simulink model "VFlexP"  (R2025a)
settings: Solver=ode23tb  StartTime=0.0  StopTime=40  FixedStep=5e-5
model workspace (MAT data in the model file):
  DCop_DCBUCK : object (value not decoded)
  Grid_CCVSC_idx = [2; 3; 4; 5; 6; 7; 8; 9; 10; 11; 12]
  Grid_CCVSCs = 1
  Grid_CCVSCs_buses = 1
  Grid_CCVSCs_toM = [0 1 0 0 0 0 0 0 0 0 0 0 ... (781 elements, 71x11)]
  Grid_C_Lines = [0.1 0.1 0.1 0.1]
  Grid_Cbuses = [0.05000002 0.10000002 0.10000002 0.10000002 0.05000002]
  Grid_DC : object (value not decoded)
  Grid_DCop_DCBUCK : object (value not decoded)
  Grid_DCop_DC_PES : object (value not decoded)
  Grid_DFIGs = 1
  Grid_DFIGs_buses = 1
  Grid_DGs : string (value not decoded)
  Grid_From_buses = [1 2 4 4]
  Grid_GFls = 1
  Grid_GFls_buses = 1
  Grid_GFr_idx = [1; 2; 3]
  Grid_GFrs = 1
  Grid_GFrs_buses = 1
  Grid_GFrs_toM = [1 0 0 0 0 0 0 0 0 1 0 0 ... (15 elements, 5x3)]
  Grid_IG_idx = 1
  Grid_IGs = 1
  Grid_IGs_buses = 1
  Grid_IGs_toM = [1; 0]
  Grid_L_Lines = [0.5 0.5 0.5 0.5]
  Grid_L_Loads = [0.000959999944704 0.000156249997559 0.00154855477548]
  Grid_Lines_fromM : object (value not decoded)
  Grid_Lines_toM : object (value not decoded)
  Grid_Load_buses = [2; 3; 4]
  Grid_Load_busesDC = []
  Grid_MGES_idx = [1; 2; 3]
  Grid_MGESs = 1
  Grid_MGESs_buses = [1; 5; 3]
  Grid_MGESs_toM = [1 0 0 0 0 0 0 0 0 1 0 0 ... (15 elements, 5x3)]
  Grid_MSGs = 1
  Grid_MSGs_buses = 1
  Grid_Nbuses = 5
  Grid_PQ_gen = [3; 2; 2]
  Grid_Ploads = [1250 4000 1250]
  Grid_PloadsDC = []
  Grid_Ps_lf = [0.274439537683 0.78 0.3]
  Grid_Qloads = [0.3 0.5 0.5]
  Grid_Qs_lf = [-0.0366071562958 0.126505596722 -0.0162964024532]
  Grid_R_Lines = [0.01 0.01 0.01 0.01]
  Grid_R_Loads = [3.9999997696 1.24999998047 3.8713869387]
  Grid_R_Loads_DC = 0
  Grid_Rcf = [50000000 50000000 50000000 50000000 50000000]
  Grid_SCs = 1
  Grid_SCs_buses = 1
  Grid_SG_idx = 1
  Grid_SGs = 1
  Grid_SGs_buses = 1
  Grid_SGs_toM = [1; 0]
  Grid_To_buses = [2 3 3 5]
  Grid_VCVSC_idx = [1; 2; 3; 4; 5; 6; 7; 8; 9; 10; 11; 12]
  Grid_VCVSCs = 1
  Grid_VCVSCs_buses = [1; 2; 3; 6; 8; 9; 12; 58; 59; 60; 63; 65]
  Grid_VCVSCs_toM = [1 0 0 0 0 0 0 0 0 0 0 0 ... (852 elements, 71x12)]
  Grid_VSM_idx = [1; 2; 3]
  Grid_VSMs = 1
  Grid_VSMs_buses = 1
  Grid_VSMs_toM = [1 0 0 0 0 0 0 0 0 1 0 0 ... (15 elements, 5x3)]
  Grid_admitt_matrix = [2.15353135314-19.7953135314i  -1.9801980198+19.801980198i; -1.9801980198+19.801980198i  2.15353135314-19.7953135314i]
  Grid_admitt_matrix_noloads = [1.98686468647-19.7953135314i  -1.9801980198+19.801980198i; -1.9801980198+19.801980198i  1.98686468647-19.7953135314i]
  Grid_bus = [1; 2; 6; 7; 8]
  Grid_busDC_complexity = [1 1 1]
  Grid_busDC_complexity_PF = [2 2 2]
  Grid_bus_complexity = [1 1 1 1 1]
  Grid_bus_complexity_PF = [1 1 1 1 1]
  Grid_buses_lf = [1; 5; 3]
  Grid_conductance_matrix = [100.00000002  -100  0; -100  200.00000002  -100; 0  -100  100.00000002]
  Grid_conductance_matrix_noloads = [100.00000002  -100  0; -100  200.00000002  -100; 0  -100  100.00000002]
  Grid_fref : object (value not decoded)
  Grid_gen_static_params : mBase (value not decoded)
  Grid_iPs_lf = [3.64378984326 1.28205128205 3.33333333333]
  Grid_iQs_lf = [-27.3170631425 7.90478860943 -61.3632366329]
  Grid_iadmitt_matrix = [2.88165849328-0.0982918688642i  2.87905051706-0.123273862303i; 2.87905051706-0.123273862303i  2.88165849328-0.0982918688642i]
  Grid_iadmitt_matrix_noloads = [37.5012524798-37.4874983544i  37.4987475202-37.5125016456i; 37.4987475202-37.5125016456i  37.5012524798-37.4874983544i]
  Grid_iconductance_matrix = [16666671.4556  16666671.4489  16666671.4456; 16666671.4489  16666671.4522  16666671.4489; 16666671.4456  16666671.4489  16666671.4556]
  Grid_iconductance_matrix_noloads = [16666671.4556  16666671.4489  16666671.4456; 16666671.4489  16666671.4522  16666671.4489; 16666671.4456  16666671.4489  16666671.4556]
  Grid_init_OK_bool = 1
  Grid_intconv_PF : object (value not decoded)
  Grid_lf_op : op_report (value not decoded)
  Grid_lineDC_complexity = [1 1]
  Grid_lineDC_complexity_PF = [2 2]
  Grid_line_complexity = [1 1 1 1]
  Grid_line_complexity_PF = [3 3 3 3]
  Grid_loadDC_complexity = []
  Grid_loadDC_complexity_PF = []
  Grid_load_complexity = [3 3 3]
  Grid_load_complexity_PF = [4 4 4]
  Grid_opDC_CCVSC : object (value not decoded)
  Grid_opDC_VSM : object (value not decoded)
  Grid_opGFr : object (value not decoded)
  Grid_opVCVSC : object (value not decoded)
  Grid_op_CCVSC : object (value not decoded)
  Grid_op_IG : object (value not decoded)
  Grid_op_MGES : object (value not decoded)
  Grid_op_SG : object (value not decoded)
  Grid_op_VSM : object (value not decoded)
  Grid_shift_lines = [0 0 0 0]
  Grid_tap_lines = [1 1 1 1]
  Grid_v_buses_mod = [1 1 1 0.9837920967 1]
  LinsysParamChangeStruct : Param1 (value not decoded)
  Lline = 0.01
  Rline = 1e-05
  linsys : object (value not decoded)
symbols that are objects in the model workspace (value not decoded): Grid_DCop_DC_PES, Grid_DCop_DCBUCK, Grid_op_CCVSC, Grid_op_IG, Grid_op_MGES, Grid_op_SG, Grid_op_VSM, Grid_opDC_CCVSC, Grid_opDC_VSM, Grid_opGFr, Grid_opVCVSC
undefined symbols (not defined in the file): block_buses_DC, block_idx, CCVSC_idx, Cf, costs, costs2, D, DFIGs_nodes, DiscIntNeverNeededParam, entity, Fb, Fi, From_nodes, grid_linsys, Grid_op_DFIG, Grid_op_DFIG_PQ, Grid_op_MSG, Grid_op_SC, Grid_op_VCVSC, H, initial_states_grid, K_1, K_3, K_5, K_A, K_C, K_IM, K_IR, K_P, K_PM, K_PR, K_S1, K_S2, K_S3, Ki_w, Kic, Kiv, Kp_id, Kp_theta, Kp_w, Kpc, Kpv, last_send, Lc, Lf, Lfd, Lkd1, Lkd2, Lkq1, Lkq2, Lkq3, Lmd, Lmq, Lsd, Lsq, m, M, Matrix_flux_to_i, mp, MSGs_buses ... (+44)
libraries: simulink x1048, eeGeneralControl x12
(part 28 of 50)

== system VFlexP/Grid/Generators/MSG/Stator circuit MSG/Subsystem2 ==
  vad : Inport
  vaq : Inport  Port=2
  id : Inport  Port=3
  iq : Inport  Port=4
  ws : Inport  Port=5
  vd : Inport  Port=6
  vq : Inport  Port=7
  Gain1 : Gain  Gain=Ra_pu
  Gain6 : Gain  Gain=Ra_pu
  Gain7 : Gain  Gain=-1
  Product{1..4} (4 alike) : Product
  Selector1 : Selector  InputPortWidth=length(fref.ref_units)  IndexOptions=Index vector (dialog)  Indices=block_fref  OutputSizes=1
  Sum1 : Sum  Inputs=-|+|-|-  InputSameDT=on  SaturateOnIntegerOverflow=on  OutDataTypeStr=Inherit: Same as first input
  Sum2 : Sum  Inputs=-|+|-|-  InputSameDT=on  SaturateOnIntegerOverflow=on  OutDataTypeStr=Inherit: Same as first input
  psis_d : Integrator  InitialCondition=Grid_op_MSG.op.States(6).x'
  psis_q : Integrator  InitialCondition=Grid_op_MSG.op.States(7).x'
  d : Outport
  q : Outport  Port=2
  wires:
  vaq/1 -> Sum2/3
  Product1/1 -> Sum2/1
  vq/1 -> Sum2/2
  Gain6/1 -> Sum2/4
  vad/1 -> Sum1/4
  vd/1 -> Sum1/2
  ws/1 -> Product1/1, Product2/2
  Product3/1 -> psis_q/1
  Product4/1 -> psis_d/1
  Gain1/1 -> Sum1/1
  psis_q/1 -> Gain7/1, q/1
  id/1 -> Gain1/1
  Product2/1 -> Sum1/3
  iq/1 -> Gain6/1
  Sum1/1 -> Product4/1
  Sum2/1 -> Product3/2
  psis_d/1 -> Product1/2, d/1
  Gain7/1 -> Product2/1
  Selector1/1 -> Product3/1, Product4/2
  [omega_base] -> Selector1/1

== system VFlexP/Grid/Generators/MSG/Subsystem/PI omega ==
  in : Inport
  Gain : Gain  Gain=KPomegar
  Gain1 : Gain  Gain=KIomegar
  Sum : Sum  Inputs=++|
  omegar : Integrator  InitialCondition=Grid_op_MSG.op.States(11).x'
  out : Outport  VectorParamsAs1DForOutWhenUnconnected=off
  wires:
  omegar/1 -> Sum/2
  Gain/1 -> Sum/1
  in/1 -> Gain/1, Gain1/1
  Sum/1 -> out/1
  Gain1/1 -> omegar/1

== system VFlexP/Grid/Generators/MSG/Vc control/PI Vc2 ==
  in : Inport
  Gain : Gain  Gain=Kp_vc2
  Gain1 : Gain  Gain=Ki_vc2
  Sum : Sum  Inputs=++|
  xa3 : Integrator  InitialCondition=Grid_op_MSG.op.States(12).x'
  out : Outport  VectorParamsAs1DForOutWhenUnconnected=off
  wires:
  Gain1/1 -> xa3/1
  Sum/1 -> out/1
  in/1 -> Gain/1, Gain1/1
  Gain/1 -> Sum/1
  xa3/1 -> Sum/2

== system VFlexP/Grid/Generators/SG/Electromagnetic/order 2 ==
  vsd : Inport
  vsq : Inport  Port=2
  ws : Inport  Port=3
  Gain : Gain  Gain=1./Lssd_pu
  Gain1 : Gain  Gain=Rs_pu
  Gain17 : Gain  Gain=-1
  Gain2 : Gain  Gain=Rs_pu
  Gain3 : Gain  Gain=1./Lssd_pu
  Gain4 : Gain
  Gain5 : Gain
  Gain6 : Gain  Gain=-1
  Gain7 : Gain  Gain=-1
  Integrator : Integrator  InitialCondition=Grid_op_SG.op.States(1).x'
  Matrix Concatenate : Concatenate  Mode=Multidimensional array
  Product{1..4} (4 alike) : Product
  Scope : Scope  NumInputPorts=2
      settings: ActiveDisplayYMinimum=-176.647  ActiveDisplayYMaximum=19.6557
  Selector2 : Selector  InputPortWidth=length(fref.ref_units)  IndexOptions=Index vector (dialog)  Indices=block_fref  OutputSizes=1
  Sum : Sum  Inputs=|++
  Sum1 : Sum  Inputs=-|+|-  InputSameDT=on  SaturateOnIntegerOverflow=on  OutDataTypeStr=Inherit: Same as first input
  Sum2 : Sum  Inputs=-|+|-  InputSameDT=on  SaturateOnIntegerOverflow=on  OutDataTypeStr=Inherit: Same as first input
  psis_d : Integrator  InitialCondition=Grid_op_SG.op.States(2).x'
  psis_q : Integrator  InitialCondition=Grid_op_SG.op.States(3).x'
  isd : Outport  VectorParamsAs1DForOutWhenUnconnected=off
  isq : Outport  Port=2  VectorParamsAs1DForOutWhenUnconnected=off
  psi : Outport  Port=3  VectorParamsAs1DForOutWhenUnconnected=off
  wires:
  Product4/1 -> Scope/1, psis_d/1
  vsd/1 -> Sum2/2
  ws/1 -> Product1/1, Product2/2
  Matrix Concatenate/1 -> psi/1
  Product3/1 -> psis_q/1
  Sum1/1 -> Product3/1
  Product1/1 -> Sum2/1
  Product2/1 -> Sum1/3
  Sum2/1 -> Product4/2
  psis_q/1 -> Sum/1, Matrix Concatenate/2, Gain17/1  "psis_q"
  Gain1/1 -> Sum1/1
  [omega_base] -> Selector2/1
  vsq/1 -> Sum1/2
  Gain/1 -> Gain4/1, Gain6/1
  Gain2/1 -> Sum2/3
  Gain3/1 -> Gain5/1, Gain7/1
  Gain17/1 -> Product1/2
  Selector2/1 -> Product4/1, Product3/2
  Sum/1 -> Gain3/1
  Integrator/1 -> Sum/2
  Gain4/1 -> Gain2/1
  Gain5/1 -> Gain1/1
  psis_d/1 -> Product2/1, Matrix Concatenate/1, Gain/1, Scope/2
  Gain6/1 -> isd/1
  Gain7/1 -> isq/1

== system VFlexP/Grid/Generators/SG/Electromagnetic/order 8 ==
  vsd : Inport
  vsq : Inport  Port=2
  vfd : Inport  Port=3
  ws : Inport  Port=4
  Stator circuit : Subsystem
  psi->i : Subsystem
  isd : Outport
  isq : Outport  Port=2
  psi : Outport  Port=3
  wires:
  psi->i/3(isq) -> isq/1
  psi->i/2(i) -> Stator circuit/3(i)
  vsd/1 -> Stator circuit/1(vsd)
  vsq/1 -> Stator circuit/2(vsq)
  ws/1 -> Stator circuit/4(ws)
  Stator circuit/1(psi) -> psi/1, psi->i/1(psi)
  vfd/1 -> Stator circuit/5(vfd)
  psi->i/1(isd) -> isd/1

== system VFlexP/Grid/Generators/SG/Electromagnetic/order 8 nomatrix ==
  vsd : Inport
  vsq : Inport  Port=2
  vfd : Inport  Port=3
  ws : Inport  Port=4
  Assignment : Assignment  NumberOfDimensions=2  DiagnosticForDimensions=Warning  IndexOptions=Index vector (dialog),Assign all  Indices=2,1  OutputSizes=1,1
  Constant : Constant  Value=Lfd_pu  VectorParams1D=off
  Integrator : Integrator  InitialCondition=Grid_op_SG.op.States(5).x'
  Selector : Selector  NumberOfDimensions=2  InputPortWidth=3  IndexOptions=Index vector (dialog),Select all  Indices=2,1  OutputSizes=1,1
  Stator circuit : Subsystem
  Sum3 : Sum  Inputs=++|
  Switch6 : Switch  Criteria=u2 ~= 0  SaturateOnIntegerOverflow=off  InputSameDT=off
  psi->i : Subsystem
  isd : Outport
  isq : Outport  Port=2
  psi : Outport  Port=3
  wires:
  psi->i/3(isq) -> isq/1
  psi->i/2(i) -> Stator circuit/3(i)
  vsd/1 -> Stator circuit/1(vsd)
  vsq/1 -> Stator circuit/2(vsq)
  ws/1 -> Stator circuit/4(ws)
  Stator circuit/1(psi) -> psi/1, Selector/1, Assignment/1
  vfd/1 -> Stator circuit/5(vfd)
  psi->i/1(isd) -> isd/1
  Sum3/1 -> Switch6/3
  Constant/1 -> Switch6/2
  Integrator/1 -> Sum3/2
  Assignment/1 -> psi->i/1(psi)
  Selector/1 -> Sum3/1, Switch6/1
  Switch6/1 -> Assignment/2

== system VFlexP/Grid/Generators/VSM/PC/LPF_P ==
  P : Inport
  Gain : Gain  Gain=100
  I : Integrator  InitialCondition=Grid_op_VSM.op.States(5).x'
  Sum4 : Sum  Inputs=|+-
  P_f : Outport
  wires:
  I/1 -> Sum4/2, P_f/1
  P/1 -> Sum4/1
  Sum4/1 -> Gain/1
  Gain/1 -> I/1

== system VFlexP/Grid/Generators/VSM/PC/LPF_Q ==
  Q : Inport
  Gain : Gain  Gain=10
  I : Integrator  InitialCondition=Grid_op_VSM.op.States(6).x'
  Sum4 : Sum  Inputs=|+-
  Q_f : Outport
  wires:
  Sum4/1 -> Gain/1
  I/1 -> Sum4/2, Q_f/1
  Q/1 -> Sum4/1
  Gain/1 -> I/1

== system VFlexP/Grid/Generators/VSM/PC/Turbine model ==
  In1 : Inport
  Out1 : Outport
  wires:
  In1/1 -> Out1/1

== system VFlexP/Grid/Generators/VSM/PC/WOF_d ==
  In1 : Inport
  Gain : Gain  Gain=10
  Gain1 : Gain  Gain=10
  I : Integrator  InitialConditionSource=external  InitialCondition=Grid_op_VSM.op.States(7).x'
  Sum : Sum  Inputs=+-|
  Sum4 : Sum  Inputs=|+-
  Out1 : Outport
  wires:
  Gain/1 -> I/1
  Sum4/1 -> Gain/1
  In1/1 -> I/2, Sum/1, Sum4/1
  I/1 -> Sum/2, Sum4/2
  Sum/1 -> Gain1/1
  Gain1/1 -> Out1/1

== system VFlexP/Grid/Generators/VSM/RL out/dynamic ==
  v_in_d : Inport
  v_out_d : Inport  Port=2
  v_in_q : Inport  Port=3
  v_out_q : Inport  Port=4
  Gain1 : Gain  Gain=L
  Gain2 : Gain  Gain=R
  Gain3 : Gain  Gain=R
  Gain4 : Gain  Gain=L
  Gain5 : Gain  Gain=invL
  Gain7 : Gain  Gain=invL
  Product{,1..3} (4 alike) : Product
  Selector7 : Selector  InputPortWidth=length(fref.ref_units)  IndexOptions=Index vector (dialog)  Indices=block_fref  OutputSizes=1
  Selector8 : Selector  InputPortWidth=length(fref.ref_units)  IndexOptions=Index vector (dialog)  Indices=block_fref  OutputSizes=1
  Sum4 : Sum  Inputs=+-|
  Sum5 : Sum  Inputs=|-+
  Sum6 : Sum  Inputs=|++
  Sum7 : Sum  Inputs=-+|
  Sum8 : Sum  Inputs=|+-
  Sum9 : Sum  Inputs=-+|
  i_d : Integrator  InitialCondition=Grid_op_VSM.op.States(7).x'
  i_q : Integrator  InitialCondition=Grid_op_VSM.op.States(8).x'
  id : Outport
  iq : Outport  Port=2
  v_outd : Outport  Port=3
  v_outq : Outport  Port=4
  wires:
  v_in_q/1 -> Sum5/2  "v_in_q"
  v_in_d/1 -> Sum4/1  "v_in_d"
  Gain2/1 -> Sum4/2
  i_d/1 -> id/1, Gain1/1, Gain2/1  "id"
  Sum6/1 -> Gain5/1
  [omega_ref] -> Selector7/1  "omega"
  Product/1 -> Sum6/2
  Sum8/1 -> Gain7/1
  Sum4/1 -> Sum7/2
  Product1/1 -> Sum8/2
  Gain4/1 -> Product/1
  Sum7/1 -> Sum6/1
  Gain3/1 -> Sum5/1
  Sum5/1 -> Sum9/2
  i_q/1 -> Gain3/1, Gain4/1, iq/1  "iq"
  Gain1/1 -> Product1/2
  Sum9/1 -> Sum8/1
  v_out_d/1 -> Sum7/1, v_outd/1  "v_out_d"
  v_out_q/1 -> Sum9/1, v_outq/1  "v_out_q"
  Selector7/1 -> Product1/1, Product/2
  [omega_base] -> Selector8/1
  Selector8/1 -> Product2/1, Product3/2
  Product3/1 -> i_d/1
  Gain5/1 -> Product3/1
  Product2/1 -> i_q/1
  Gain7/1 -> Product2/2

== system VFlexP/Grid/Generators/VSM/RL out/static ==
  v_in_d : Inport
  v_out_d : Inport  Port=2
  v_in_q : Inport  Port=3
  v_out_q : Inport  Port=4
  Constant : Constant  Value=R.^2
  Constant1 : Constant
  Divide : Product  Inputs=*/
  Gain : Gain  Gain=L
  Gain1 : Gain  Gain=R
  Gain2 : Gain  Gain=R
  Product{,1..5} (6 alike) : Product
  Selector7 : Selector  InputPortWidth=length(fref.ref_units)  IndexOptions=Index vector (dialog)  Indices=block_fref  OutputSizes=1
  Sum : Sum  Inputs=|++
  Sum1 : Sum  Inputs=|+-
  Sum2 : Sum  Inputs=|+-
  Sum3 : Sum  Inputs=|++
  Sum4 : Sum  Inputs=|-+
  id : Outport
  iq : Outport  Port=2
  v_outd : Outport  Port=3
  v_outq : Outport  Port=4
  wires:
  v_in_q/1 -> Sum2/1  "v_in_q"
  v_out_d/1 -> Sum1/2, v_outd/1  "v_out_d"
  Sum/1 -> Divide/2
  Gain2/1 -> Product5/2
  Product/1 -> Sum/2
  Product1/1 -> Sum3/1
  Product5/1 -> Sum4/2
  Constant/1 -> Sum/1
  Sum2/1 -> Product3/2, Product5/1  "vq"
  Gain/1 -> Product2/2, Product/1, Product/2
  Constant1/1 -> Divide/1
  Product3/1 -> Sum3/2
  Sum1/1 -> Product4/1, Product1/1  "vd"
  Divide/1 -> Product2/1, Gain1/1, Gain2/1
  Product4/1 -> Sum4/1
  Product2/1 -> Product3/1, Product4/2
  Gain1/1 -> Product1/2
  Sum3/1 -> id/1  "id"
  Sum4/1 -> iq/1  "iq"
  v_out_q/1 -> Sum2/2, v_outq/1  "v_out_q"
  v_in_d/1 -> Sum1/1  "v_in_d"
  [omega_ref] -> Selector7/1  "omega"
  Selector7/1 -> Gain/1

== system VFlexP/Grid/Generators/VSM/RL out/static_omega ==
  v_in_d : Inport
  v_out_d : Inport  Port=2
  v_in_q : Inport  Port=3
  v_out_q : Inport  Port=4
  Gain : Gain  Gain=1./(R.^2+L.^2)
  Gain2 : Gain  Gain=1./(R.^2+L.^2)
  Gain3 : Gain  Gain=R
  Gain4 : Gain  Gain=L
  Gain5 : Gain  Gain=L
  Gain6 : Gain  Gain=R
  Sum : Sum  Inputs=|++
  Sum1 : Sum  Inputs=|+-
  Sum2 : Sum  Inputs=|+-
  Sum3 : Sum  Inputs=|-+
  id : Outport
  iq : Outport  Port=2
  v_outd : Outport  Port=3
  v_outq : Outport  Port=4
  wires:
  Gain6/1 -> Sum3/2
  Sum3/1 -> iq/1
  Gain5/1 -> Sum3/1
  Sum/1 -> id/1
  Gain2/1 -> Gain4/1, Gain6/1
  Gain4/1 -> Sum/2
  Gain3/1 -> Sum/1
  Gain/1 -> Gain3/1, Gain5/1
  Sum2/1 -> Gain2/1  "vq"
  Sum1/1 -> Gain/1  "vd"
  v_out_d/1 -> Sum1/2, v_outd/1  "v_out_d"
  v_out_q/1 -> Sum2/2, v_outq/1  "v_out_q"
  v_in_d/1 -> Sum1/1  "v_in_d"
  v_in_q/1 -> Sum2/1  "v_in_q"

== system VFlexP/Grid/Generators/VSM/VCC/dynamic ==
  vodref : Inport
  voqref : Inport  Port=2
  iod : Inport  Port=3
  ioq : Inport  Port=4
  omega : Inport  Port=5
  Cf : Gain  Gain=Cfi
  Cf 1 : Gain  Gain=Cfi
  Fi : Gain  Gain=Fi
  Fi2 : Gain  Gain=Fi
  "Lf " : Gain  Gain=Lf
  Lf1 : Gain  Gain=Lf
  Product{,1..3} (4 alike) : Product
  RC : Subsystem  Variant=on  VariantControlMode=label  LabelModeActiveChoice=dynamic  mask{dynamic=Dynamic, R=Rcf, C=Cfi, fbase=50}
      mask prompts: dynamic "Dynamic behavior"; R "Parallel resistance (p.u.)"; C "Capacitance (p.u.)"; fbase "Base frequency (Hz)"
      mask init: same as VFlexP/Grid/DCAC converters/DC_VCVSC/VCC/dynamic/RC
      mask TypeOptions dynamic: Dynamic | Static | Static omega
  RL : Subsystem  Variant=on  VariantControlMode=label  LabelModeActiveChoice=dynamic  mask(Line){dynamic=Dynamic, R=Rf, L=Lf, fbase=50}
      mask prompts: dynamic "Dynamic behavior"; R "Series resistance (p.u.)"; L "Inductance (p.u.)"; fbase "Base frequency (Hz)"
      mask init: same as VFlexP/Grid/DCAC converters/DC_VCVSC/RL out
      mask Help: web('Documentation/RL.html')
      mask TypeOptions dynamic: Static | Dynamic | Static omega
  Subsystem : Subsystem
  Subsystem1 : Subsystem
  Subsystem2 : Subsystem
  Subsystem3 : Subsystem
  Sum1 : Sum  Inputs=++|
  Sum2 : Sum  Inputs=-+|
  Sum{3,5..6,9} (4 alike) : Sum  Inputs=|++
  Sum4 : Sum  Inputs=++|
  Sum8 : Sum  Inputs=-+|
  vidref : Outport
  viqref : Outport  Port=2
  wires:
  Sum6/1 -> RL/3(v_in_q)
  Sum1/1 -> RL/1(v_in_d)
  Sum9/1 -> Sum6/1  "viqref"
  Sum8/1 -> Sum1/2  "vidref"
  RL/2(iq) -> "Lf "/1, Subsystem3/2(y), RC/3(i_q_in)
  RL/1(id) -> RC/1(i_d_in), Lf1/1, Subsystem2/2(y)
  RC/1(v_d) -> Cf 1/1, Subsystem/2(y), RL/2(v_out_d), Sum1/1, vidref/1
  [omega] -> Product1/1
  omega/1 -> [omega], Product2/1  "omega"
  Subsystem3/1(Out1) -> Sum9/1
  Subsystem2/1(Out1) -> Sum8/2
  Subsystem1/1(Out1) -> Sum3/1
  Subsystem/1(Out1) -> Sum2/2
  Fi2/1 -> Sum5/2
  ioq/1 -> Fi2/1, RC/4(i_q_out)  "ioq"
  [omega] -> Product3/1, RC/5(omega)  "omega"
  Sum3/1 -> Sum5/1
  "Lf "/1 -> Product/1
  Sum2/1 -> Sum4/2
  iod/1 -> Fi/1, RC/2(i_d_out)  "iod"
  Product1/1 -> Sum2/1
  Sum4/1 -> Subsystem2/1(ref)  "ildref"
  Cf/1 -> Product1/2
  Cf 1/1 -> Product2/2
  Product2/1 -> Sum3/2
  Product3/1 -> Sum9/2
  voqref/1 -> Subsystem1/1(ref)  "voqref"
  Fi/1 -> Sum4/1
  Lf1/1 -> Product3/2
  [omega] -> Product/2
  RC/2(v_q) -> Cf/1, Subsystem1/2(y), RL/4(v_out_q), Sum6/2, viqref/1  "voq"
  vodref/1 -> Subsystem/1(ref)  "vodref"
  Product/1 -> Sum8/1
  Sum5/1 -> Subsystem3/1(ref)  "ilqref"

== system VFlexP/Grid/Generators/VSM/VCC/dynamic_VC ==
  vodref : Inport
  voqref : Inport  Port=2
  iod : Inport  Port=3
  ioq : Inport  Port=4
  omega : Inport  Port=5
  Cf : Gain  Gain=Cfi
  Cf 1 : Gain  Gain=Cfi
  Fi : Gain  Gain=Fi
  Fi2 : Gain  Gain=Fi
  Product1 : Product
  Product2 : Product
  RC : Subsystem  Variant=on  VariantControlMode=label  LabelModeActiveChoice=dynamic  mask{dynamic=Dynamic, R=Rcf, C=Cfi, fbase=Fb}
      mask prompts: dynamic "Dynamic behavior"; R "Parallel resistance (p.u.)"; C "Capacitance (p.u.)"; fbase "Base frequency (Hz)"
      mask init: same as VFlexP/Grid/DCAC converters/DC_VCVSC/VCC/dynamic/RC
      mask TypeOptions dynamic: Dynamic | Static | Static omega
  Subsystem : Subsystem
  Subsystem1 : Subsystem
  Sum2 : Sum  Inputs=-+|
  Sum3 : Sum  Inputs=|++
  Sum4 : Sum  Inputs=++|
  Sum5 : Sum  Inputs=|++
  vidref : Outport
  viqref : Outport  Port=2
  wires:
  Sum5/1 -> RC/3(i_q_in)
  Sum4/1 -> RC/1(i_d_in)
  RC/1(v_d) -> Subsystem/2(y), Cf 1/1, vidref/1
  vodref/1 -> Subsystem/1(ref)  "vodref"
  RC/2(v_q) -> Subsystem1/2(y), Cf/1, viqref/1
  Fi/1 -> Sum4/1
  voqref/1 -> Subsystem1/1(ref)  "voqref"
  Product2/1 -> Sum3/2
  Cf 1/1 -> Product2/2
  Cf/1 -> Product1/2
  Product1/1 -> Sum2/1
  iod/1 -> Fi/1, RC/2(i_d_out)  "iod"
  Sum2/1 -> Sum4/2
  Sum3/1 -> Sum5/1
  ioq/1 -> Fi2/1, RC/4(i_q_out)  "ioq"
  Fi2/1 -> Sum5/2
  Subsystem/1(Out1) -> Sum2/2
  Subsystem1/1(Out1) -> Sum3/1
  omega/1 -> [omega], Product2/1, RC/5(omega)  "omega"
  [omega] -> Product1/1

== system VFlexP/Grid/Generators/VSM/VCC/dynamic_limiting ==
  note: Current limiting, no priority
  vodref : Inport
  voqref : Inport  Port=2
  iod : Inport  Port=3
  ioq : Inport  Port=4
  omega : Inport  Port=5
  Abs : Abs  ZeroCross=off  SaturateOnIntegerOverflow=off
  Abs1 : Abs  ZeroCross=off  SaturateOnIntegerOverflow=off
  Abs2 : Abs  ZeroCross=off  SaturateOnIntegerOverflow=off
  Cf : Gain  Gain=Cfi
  Cf 1 : Gain  Gain=Cfi
  Divide : Product  Inputs=*/
  Divide1 : Product  Inputs=*/
  Fi : Gain  Gain=Fi
  Fi2 : Gain  Gain=Fi
  Gain : Gain  Gain=-1
  Gain1 : Gain  Gain=-1
  "Lf " : Gain  Gain=Lf
  Lf1 : Gain  Gain=Lf
  Memory : Memory  InitialCondition=1  LinearizeMemory=on
  Memory1 : Memory  InitialCondition=1  LinearizeMemory=on
  PIi_d : Subsystem
  PIi_q : Subsystem
  PIv_d : Subsystem
  PIv_q : Subsystem
  Product{,1..3} (4 alike) : Product
  RC : Subsystem  Variant=on  VariantControlMode=label  LabelModeActiveChoice=dynamic  mask{dynamic=Dynamic, R=Rcf, C=Cfi, fbase=Fb}
      mask prompts: dynamic "Dynamic behavior"; R "Parallel resistance (p.u.)"; C "Capacitance (p.u.)"; fbase "Base frequency (Hz)"
      mask init: same as VFlexP/Grid/DCAC converters/DC_VCVSC/VCC/dynamic/RC
      mask TypeOptions dynamic: Dynamic | Static | Static omega
  RL : Subsystem  Variant=on  VariantControlMode=label  LabelModeActiveChoice=dynamic  mask(Line){dynamic=Dynamic, R=Rf, L=Lf, fbase=Fb}
      mask prompts: dynamic "Dynamic behavior"; R "Series resistance (p.u.)"; L "Inductance (p.u.)"; fbase "Base frequency (Hz)"
      mask init: same as VFlexP/Grid/DCAC converters/DC_VCVSC/RL out
      mask Help: web('Documentation/RL.html')
      mask TypeOptions dynamic: Static | Dynamic | Static omega
  Real-Imag to Complex : RealImagToComplex
  Relational Operator : RelationalOperator  Operator===  OutDataTypeStr=boolean  ZeroCross=off  RndMeth=Simplest  InputSameDT=off
  Relational Operator1 : RelationalOperator  Operator===  OutDataTypeStr=boolean  ZeroCross=off  RndMeth=Simplest  InputSameDT=off
  Saturation Dynamic : simulink/Discontinuities/Saturation Dynamic  OutMin=[]  OutMax=[]  OutDataTypeStr=Inherit: Same as second input  OutDataType=fixdt(1, 16)  OutScaling=2^-10  DoSatur=off
  Saturation Dynamic1 : simulink/Discontinuities/Saturation Dynamic  OutMin=[]  OutMax=[]  OutDataTypeStr=Inherit: Same as second input  OutDataType=fixdt(1, 16)  OutScaling=2^-10  DoSatur=off
  Sum : Sum  Inputs=|+-
  Sum{1..2,6,8} (4 alike) : Sum  Inputs=-+|
  Sum3 : Sum  Inputs=|++
  Sum4 : Sum  Inputs=++|
  Sum5 : Sum  Inputs=|++
  Sum7 : Sum  Inputs=|+-
  Sum9 : Sum  Inputs=|++
  vidref : Outport
  viqref : Outport  Port=2
  wires:
  Memory/1 -> PIv_d/2(In2)
  Memory1/1 -> PIv_q/2(In2)
  Relational Operator1/1 -> Memory1/1
  Sum/1 -> PIv_q/1(In1)
  Relational Operator/1 -> Memory/1
  Sum1/1 -> PIv_d/1(In1)
  Gain1/1 -> Saturation Dynamic/3
  Gain/1 -> Saturation Dynamic1/3
  Divide1/1 -> Saturation Dynamic1/1, Gain/1
  Divide/1 -> Saturation Dynamic/1, Gain1/1
  Abs/1 -> Divide/2, Divide1/2
  Real-Imag to Complex/1 -> Abs/1
  Sum5/1 -> Real-Imag to Complex/2, Saturation Dynamic1/2, Abs1/1, Relational Operator1/1  "ilqref"
  Product/1 -> Sum8/1
  vodref/1 -> Sum1/2  "vodref"
  RC/2(v_q) -> viqref/1, RL/4(v_out_q), Sum/2, Cf/1  "voq"
  [omega] -> Product/2
  Lf1/1 -> Product3/2
  Fi/1 -> Sum4/1
  Sum6/1 -> PIi_d/1(In1)
  voqref/1 -> Sum/1  "voqref"
  Product3/1 -> Sum9/2
  Product2/1 -> Sum3/2
  Cf 1/1 -> Product2/2
  Cf/1 -> Product1/2
  Sum4/1 -> Real-Imag to Complex/1, Saturation Dynamic/2, Abs2/1, Relational Operator/1  "ildref"
  Product1/1 -> Sum2/1
  iod/1 -> RC/2(i_d_out), Fi/1  "iod"
  Sum2/1 -> Sum4/2
  Sum7/1 -> PIi_q/1(In1)
  "Lf "/1 -> Product/1
  Sum3/1 -> Sum5/1
  [omega] -> RC/5(omega), Product3/1  "omega"
  ioq/1 -> RC/4(i_q_out), Fi2/1  "ioq"
  Fi2/1 -> Sum5/2
  PIv_d/1(Out1) -> Sum2/2
  PIv_q/1(Out1) -> Sum3/1
  PIi_d/1(Out1) -> Sum8/2
  PIi_q/1(Out1) -> Sum9/1
  omega/1 -> Product2/1, [omega]  "omega"
  [omega] -> Product1/1
  RC/1(v_d) -> vidref/1, RL/2(v_out_d), Cf 1/1, Sum1/1
  RL/1(id) -> Lf1/1, Sum6/1, RC/1(i_d_in)
  RL/2(iq) -> RC/3(i_q_in), "Lf "/1, Sum7/2
  Sum8/1 -> RL/1(v_in_d)  "vidref"
  Sum9/1 -> RL/3(v_in_q)  "viqref"
  Abs1/1 -> Divide1/1
  Abs2/1 -> Divide/1
  Saturation Dynamic1/1 -> Relational Operator1/2, Sum7/1
  Saturation Dynamic/1 -> Relational Operator/2, Sum6/2

== system VFlexP/Grid/Generators/VSM/VCC/static ==
  vodref : Inport
  voqref : Inport  Port=2
  iod : Inport  Port=3
  ioq : Inport  Port=4
  omega : Inport  Port=5
  Terminator : Terminator
  Terminator1 : Terminator
  Terminator2 : Terminator
  vidref : Outport
  viqref : Outport  Port=2
  wires:
  omega/1 -> Terminator2/1  "ioq"
  ioq/1 -> Terminator1/1  "ioq"
  iod/1 -> Terminator/1  "iod"
  vodref/1 -> vidref/1  "vodref"
  voqref/1 -> viqref/1  "voqref"

== system VFlexP/Grid/Generators/VSM/VI/WOF_d ==
  In1 : Inport
  Gain : Gain  Gain=iTf
  I : Integrator  InitialConditionSource=external  InitialCondition=Grid_op_VCVSC.op.States(6).x'
  Sum : Sum  Inputs=+-|
  Sum4 : Sum  Inputs=|+-
  Out1 : Outport
  wires:
  Gain/1 -> I/1
  Sum4/1 -> Gain/1
  In1/1 -> I/2, Sum/1, Sum4/1
  I/1 -> Sum/2, Sum4/2
  Sum/1 -> Out1/1

== system VFlexP/Grid/Generators/VSM/VI/WOF_q ==
  In1 : Inport
  Gain : Gain  Gain=iTf
  I : Integrator  InitialConditionSource=external  InitialCondition=Grid_op_VCVSC.op.States(7).x'
  Sum : Sum  Inputs=+-|
  Sum4 : Sum  Inputs=|+-
  Out1 : Outport
  wires:
  Gain/1 -> I/1
  Sum4/1 -> Gain/1
  In1/1 -> I/2, Sum/1, Sum4/1
  I/1 -> Sum/2, Sum4/2
  Sum/1 -> Out1/1

== system VFlexP/Grid/Grid/Dynamic/Buses/dynamic ==
  i_in : Inport
  i_out : Inport  Port=2
  Constant : Constant  Value=zeros(1, sum(bus_complexity == 1))  VectorParams1D=off
  Divide : Product  Inputs=*/
  Divide1 : Product  Inputs=*/
  For Each Subsystem : Subsystem  TreatAsAtomicUnit=on
  Gain1 : Gain  Gain=1./Rcf(bus_complexity == 1)
  Gain2 : Gain  Gain=1./Rcf(bus_complexity == 1)
  Matrix Concatenate : Concatenate  NumInputs=3  Mode=Multidimensional array
  Product : Product  Inputs=3
  Product1 : Product  Inputs=3
  Product2 : Product
  Product3 : Product
  Selector : Selector  NumberOfDimensions=2  InputPortWidth=3  IndexOptions=Index vector (dialog),Index vector (dialog)  Indices=1,find(bus_complexity == 1)  OutputSizes=1,1
  Selector1 : Selector  NumberOfDimensions=2  InputPortWidth=3  IndexOptions=Index vector (dialog),Index vector (dialog)  Indices=2,find(bus_complexity == 1)  OutputSizes=1,1
  Selector2 : Selector  NumberOfDimensions=2  InputPortWidth=3  IndexOptions=Index vector (dialog),Index vector (dialog)  Indices=1,find(bus_complexity == 1)  OutputSizes=1,1
  Selector3 : Selector  NumberOfDimensions=2  InputPortWidth=3  IndexOptions=Index vector (dialog),Index vector (dialog)  Indices=2,find(bus_complexity == 1)  OutputSizes=1,1
  Selector4 : Selector  InputPortWidth=length(fref.ref_units)  IndexOptions=Index vector (dialog)  Indices=fref.buses(bus_complexity == 1)  OutputSizes=1
  Selector5 : Selector  InputPortWidth=length(Cbuses)  IndexOptions=Index vector (dialog)  Indices=find(bus_complexity == 1)  OutputSizes=1
  Selector8 : Selector  InputPortWidth=length(fref.ref_units)  IndexOptions=Index vector (dialog)  Indices=fref.buses(bus_complexity == 1)  OutputSizes=1
  Signal Specification : SignalSpecification  Dimensions=[3 sum(bus_complexity == 1)]
  Sum10 : Sum  Inputs=|-++
  Sum11 : Sum  Inputs=-+|
  Sum12 : Sum  Inputs=|+-
  Sum13 : Sum  Inputs=-+-|
  vd : Integrator  InitialCondition=Grid_lf_op.op_report.Outputs(7).y(bus_complexity == 1)
  vq : Integrator  InitialCondition=Grid_lf_op.op_report.Outputs(8).y(bus_complexity == 1)
  v : Outport
  wires:
  Sum10/1 -> Divide/1
  vq/1 -> Product1/1, Gain2/1, Matrix Concatenate/2  "vq"
  Product1/1 -> Sum10/3
  Gain2/1 -> Sum13/3
  Product/1 -> Sum13/1
  Sum11/1 -> Sum10/2
  [omega_ref] -> Selector4/1  "omega"
  Gain1/1 -> Sum10/1
  Sum12/1 -> Sum13/2
  vd/1 -> Gain1/1, Matrix Concatenate/1, Product/1  "vd"
  Selector/1 -> Sum11/2  "id1"
  Selector2/1 -> Sum11/1  "id2"
  Selector1/1 -> Sum12/1  "iq1"
  Selector3/1 -> Sum12/2  "iq2"
  i_in/1 -> Selector/1, Selector1/1
  i_out/1 -> Selector3/1, Selector2/1
  Matrix Concatenate/1 -> Signal Specification/1
  For Each Subsystem/1(Out1) -> v/1
  Signal Specification/1 -> For Each Subsystem/1(In1)
  Constant/1 -> Matrix Concatenate/3
  Selector4/1 -> Product1/2, Product/2
  Divide/1 -> Product2/1
  Divide1/1 -> Product3/2
  [omega_base] -> Selector8/1
  Selector8/1 -> Product2/2, Product3/1
  Product2/1 -> vd/1
  Product3/1 -> vq/1
  [Cbuses] -> Selector5/1
  Selector5/1 -> [Cb]
  [Cb] -> Product/3
  [Cb] -> Product1/3
  [Cb] -> Divide/2
  [Cb] -> Divide1/2
  Sum13/1 -> Divide1/1

== system VFlexP/Grid/Grid/Dynamic/Buses/only R ==
  i_in : Inport
  i_out : Inport  Port=2
  Constant : Constant  Value=zeros(1, sum(bus_complexity == 4))  VectorParams1D=off
  For Each Subsystem : Subsystem  TreatAsAtomicUnit=on
  Gain : Gain  Gain=Rcf(bus_complexity == 4)
  Gain2 : Gain  Gain=Rcf(bus_complexity == 4)
  Matrix Concatenate : Concatenate  NumInputs=3  Mode=Multidimensional array
  Selector : Selector  NumberOfDimensions=2  InputPortWidth=3  IndexOptions=Index vector (dialog),Index vector (dialog)  Indices=1,find(bus_complexity == 4)  OutputSizes=1,1
  Selector1 : Selector  NumberOfDimensions=2  InputPortWidth=3  IndexOptions=Index vector (dialog),Index vector (dialog)  Indices=2,find(bus_complexity == 4)  OutputSizes=1,1
  Selector2 : Selector  NumberOfDimensions=2  InputPortWidth=3  IndexOptions=Index vector (dialog),Index vector (dialog)  Indices=1,find(bus_complexity == 4)  OutputSizes=1,1
  Selector3 : Selector  NumberOfDimensions=2  InputPortWidth=3  IndexOptions=Index vector (dialog),Index vector (dialog)  Indices=2,find(bus_complexity == 4)  OutputSizes=1,1
  Sum1 : Sum  Inputs=|+-
  Sum2 : Sum  Inputs=|+-
  v : Outport
  wires:
  Selector1/1 -> Sum2/1  "iq1"
  Sum1/1 -> Gain/1  "id"
  Sum2/1 -> Gain2/1  "iq"
  Selector3/1 -> Sum2/2  "iq2"
  Selector/1 -> Sum1/1  "id"
  Selector2/1 -> Sum1/2
  Gain2/1 -> Matrix Concatenate/2
  Gain/1 -> Matrix Concatenate/1
  i_in/1 -> Selector/1, Selector1/1
  Matrix Concatenate/1 -> For Each Subsystem/1(In1)
  i_out/1 -> Selector2/1, Selector3/1
  For Each Subsystem/1(Out1) -> v/1
  Constant/1 -> Matrix Concatenate/3

== system VFlexP/Grid/Grid/Dynamic/Buses/static ==
  i_in : Inport
  i_out : Inport  Port=2
  Constant : Constant  Value=(1./Rcf(bus_complexity == 2)).^2  VectorParams1D=off
  Constant1 : Constant
  Constant2 : Constant  Value=zeros(1, sum(bus_complexity == 2))  VectorParams1D=off
  Divide : Product  Inputs=*/
  For Each Subsystem : Subsystem  TreatAsAtomicUnit=on
  Gain1 : Gain  Gain=1./Rcf(bus_complexity == 2)
  Gain2 : Gain  Gain=1./Rcf(bus_complexity == 2)
  Matrix Concatenate : Concatenate  NumInputs=3  Mode=Multidimensional array
  Product{,1..6} (7 alike) : Product
  Selector : Selector  NumberOfDimensions=2  InputPortWidth=3  IndexOptions=Index vector (dialog),Index vector (dialog)  Indices=1,find(bus_complexity == 2)  OutputSizes=1,1
  Selector1 : Selector  NumberOfDimensions=2  InputPortWidth=3  IndexOptions=Index vector (dialog),Index vector (dialog)  Indices=2,find(bus_complexity == 2)  OutputSizes=1,1
  Selector2 : Selector  NumberOfDimensions=2  InputPortWidth=3  IndexOptions=Index vector (dialog),Index vector (dialog)  Indices=1,find(bus_complexity == 2)  OutputSizes=1,1
  Selector3 : Selector  NumberOfDimensions=2  InputPortWidth=3  IndexOptions=Index vector (dialog),Index vector (dialog)  Indices=2,find(bus_complexity == 2)  OutputSizes=1,1
  Selector4 : Selector  InputPortWidth=length(fref.ref_units)  IndexOptions=Index vector (dialog)  Indices=fref.buses(bus_complexity == 2)  OutputSizes=1
  Selector5 : Selector  InputPortWidth=length(Cbuses)  IndexOptions=Index vector (dialog)  Indices=find(bus_complexity == 2)  OutputSizes=1
  Sum : Sum  Inputs=|++
  Sum1 : Sum  Inputs=|-+
  Sum2 : Sum  Inputs=|+-
  Sum3 : Sum  Inputs=|++
  Sum4 : Sum  Inputs=|-+
  v : Outport
  wires:
  Product5/1 -> Sum4/2
  Gain2/1 -> Product5/2
  Product4/1 -> Sum4/1
  Product2/1 -> Product3/1, Product4/2
  Product3/1 -> Sum3/2
  Product1/1 -> Sum3/1
  Divide/1 -> Product2/1, Gain1/1, Product5/1
  Gain1/1 -> Product1/2
  Sum2/1 -> Product3/2, Gain2/1  "iq"
  Sum1/1 -> Product4/1, Product1/1  "id"
  Constant1/1 -> Divide/1
  Product/1 -> Sum/2
  Product6/1 -> Product/1, Product/2, Product2/2
  Sum/1 -> Divide/2
  Constant/1 -> Sum/1
  Sum4/1 -> Matrix Concatenate/2  "vq"
  Sum3/1 -> Matrix Concatenate/1  "vd"
  [omega_ref] -> Selector4/1  "omega"
  Selector/1 -> Sum1/2  "id1"
  Selector2/1 -> Sum1/1  "id2"
  Selector1/1 -> Sum2/1  "iq1"
  Selector3/1 -> Sum2/2  "iq2"
  i_in/1 -> Selector/1, Selector1/1
  Matrix Concatenate/1 -> For Each Subsystem/1(In1)
  i_out/1 -> Selector2/1, Selector3/1
  For Each Subsystem/1(Out1) -> v/1
  Constant2/1 -> Matrix Concatenate/3
  Selector4/1 -> Product6/2
  Selector5/1 -> [Cb]
  [Cbuses] -> Selector5/1
  [Cb] -> Product6/1

== system VFlexP/Grid/Grid/Dynamic/Buses/static omega ==
  i_in : Inport
  i_out : Inport  Port=2
  Constant : Constant  Value=zeros(1, sum(bus_complexity == 3))  VectorParams1D=off
  For Each Subsystem : Subsystem  TreatAsAtomicUnit=on
  Gain : Gain  Gain=1./((1./Rcf(bus_complexity == 3)).^2+Cbuses(bus_complexity == 3).^2)
  Gain1 : Gain  Gain=1./((1./Rcf(bus_complexity == 3)).^2+Cbuses(bus_complexity == 3).^2)
  Gain3 : Gain  Gain=1./Rcf(bus_complexity == 3)
  Gain5 : Gain  Gain=1./Rcf(bus_complexity == 3)
  IC : InitialCondition  Value=[Grid_lf_op.op_report.Outputs(7).y(bus_complexity == 3); Grid_lf_op.op_report.Outputs(8).y(bus_complexity == 3); 0*Grid_lf_op.op_report.Outputs(7).y(bus_complexity == 3)]
  LPF : Subsystem  Commented=through
  Matrix Concatenate : Concatenate  NumInputs=3  Mode=Multidimensional array
  Product : Product
  Product1 : Product
  Selector : Selector  NumberOfDimensions=2  InputPortWidth=3  IndexOptions=Index vector (dialog),Index vector (dialog)  Indices=1,find(bus_complexity == 3)  OutputSizes=1,1
  Selector1 : Selector  NumberOfDimensions=2  InputPortWidth=3  IndexOptions=Index vector (dialog),Index vector (dialog)  Indices=2,find(bus_complexity == 3)  OutputSizes=1,1
  Selector2 : Selector  NumberOfDimensions=2  InputPortWidth=3  IndexOptions=Index vector (dialog),Index vector (dialog)  Indices=1,find(bus_complexity == 3)  OutputSizes=1,1
  Selector3 : Selector  NumberOfDimensions=2  InputPortWidth=3  IndexOptions=Index vector (dialog),Index vector (dialog)  Indices=2,find(bus_complexity == 3)  OutputSizes=1,1
  Selector5 : Selector  InputPortWidth=length(Cbuses)  IndexOptions=Index vector (dialog)  Indices=find(bus_complexity == 3)  OutputSizes=1
  Sum : Sum  Inputs=|++
  Sum1 : Sum  Inputs=|+-
  Sum2 : Sum  Inputs=|+-
  Sum4 : Sum  Inputs=|-+
  v : Outport
  wires:
  Selector1/1 -> Sum2/1  "iq1"
  Sum1/1 -> Gain/1  "id"
  Sum2/1 -> Gain1/1  "iq"
  Selector3/1 -> Sum2/2  "iq2"
  Selector/1 -> Sum1/1  "id"
  Selector2/1 -> Sum1/2
  Gain/1 -> Product/1, Gain3/1
  Gain1/1 -> Product1/1, Gain5/1
  Gain3/1 -> Sum/1
  Product1/1 -> Sum/2
  Product/1 -> Sum4/1
  Gain5/1 -> Sum4/2
  Sum4/1 -> Matrix Concatenate/2
  Sum/1 -> Matrix Concatenate/1
  i_in/1 -> Selector1/1, Selector/1
  i_out/1 -> Selector3/1, Selector2/1
  For Each Subsystem/1(Out1) -> v/1
  Constant/1 -> Matrix Concatenate/3
  Matrix Concatenate/1 -> LPF/1(in)
  LPF/1(out) -> IC/1
  IC/1 -> For Each Subsystem/1(In1)
  Selector5/1 -> [Cb]
  [Cbuses] -> Selector5/1
  [Cb] -> Product/2
  [Cb] -> Product1/2

== system VFlexP/Grid/Grid/Dynamic/Lines/dynamic ==
  v_in_d : Inport
  v_out : Inport  Port=2
  connected : Inport  Port=3
  Constant1 : Constant  Value=zeros(1, sum(line_complexity == 1))  VectorParams1D=off
  For Each Subsystem : Subsystem  TreatAsAtomicUnit=on
  Gain1 : Gain  Gain=L_Lines(line_complexity == 1)
  Gain2 : Gain  Gain=R_Lines(line_complexity == 1)
  Gain3 : Gain  Gain=R_Lines(line_complexity == 1)
  Gain4 : Gain  Gain=L_Lines(line_complexity == 1)
  Gain5 : Gain  Gain=1./L_Lines(line_complexity == 1)
  Gain6 : Gain  Gain=1./L_Lines(line_complexity == 1)
  Matrix Concatenate : Concatenate  NumInputs=3  Mode=Multidimensional array
  Product{,1..9} (10 alike) : Product
  Selector : Selector  NumberOfDimensions=2  InputPortWidth=3  IndexOptions=Index vector (dialog),Index vector (dialog)  Indices=1,find(line_complexity == 1)  OutputSizes=1,1
  Selector1 : Selector  NumberOfDimensions=2  InputPortWidth=3  IndexOptions=Index vector (dialog),Index vector (dialog)  Indices=1,find(line_complexity == 1)  OutputSizes=1,1
  Selector2 : Selector  NumberOfDimensions=2  InputPortWidth=3  IndexOptions=Index vector (dialog),Index vector (dialog)  Indices=2,find(line_complexity == 1)  OutputSizes=1,1
  Selector3 : Selector  NumberOfDimensions=2  InputPortWidth=3  IndexOptions=Index vector (dialog),Index vector (dialog)  Indices=2,find(line_complexity == 1)  OutputSizes=1,1
  Selector4 : Selector  InputPortWidth=length(From_buses)  IndexOptions=Index vector (dialog)  Indices=find(line_complexity == 1)  OutputSizes=1
  Selector5 : Selector  InputPortWidth=length(fref.ref_units)  IndexOptions=Index vector (dialog)  Indices=fref.lines(line_complexity == 1)  OutputSizes=1
  Selector6 : Selector  InputPortWidth=length(From_buses)  IndexOptions=Index vector (dialog)  Indices=find(line_complexity == 1)  OutputSizes=1
  Selector8 : Selector  InputPortWidth=length(fref.ref_units)  IndexOptions=Index vector (dialog)  Indices=fref.lines(line_complexity == 1)  OutputSizes=1
  Signal Specification : SignalSpecification  Dimensions=[3 sum(line_complexity == 1)]
  Sum4 : Sum  Inputs=+-|
  Sum5 : Sum  Inputs=|-+
  Sum6 : Sum  Inputs=|++
  Sum7 : Sum  Inputs=-+|
  Sum8 : Sum  Inputs=|+-
  Sum9 : Sum  Inputs=-+|
  connected1 : InportShadow  Port=3
  i_d : Integrator  InitialCondition=Grid_lf_op.op_report.Outputs(3).y(line_complexity == 1)
  i_q : Integrator  InitialCondition=Grid_lf_op.op_report.Outputs(4).y(line_complexity == 1)
  i : Outport
  wires:
  v_out/1 -> Selector3/1, Selector1/1  "v_out"
  Sum9/1 -> Sum8/1
  Gain1/1 -> Product1/2
  i_q/1 -> Gain3/1, Gain4/1, Product3/2  "iq"
  Sum5/1 -> Sum9/2
  Gain3/1 -> Sum5/1
  Sum7/1 -> Sum6/1
  Gain4/1 -> Product/1
  Product1/1 -> Sum8/2
  Sum4/1 -> Sum7/2
  Sum8/1 -> Gain6/1
  Product/1 -> Sum6/2
  [omega_ref] -> Selector5/1  "omega"
  Sum6/1 -> Gain5/1
  i_d/1 -> Gain1/1, Gain2/1, Product2/2  "id"
  Gain2/1 -> Sum4/2
  v_in_d/1 -> Selector2/1, Selector/1  "v_in"
  Product5/1 -> Sum5/2
  connected/1 -> Selector4/1
  Matrix Concatenate/1 -> Signal Specification/1
  Product2/1 -> Matrix Concatenate/1
  Product3/1 -> Matrix Concatenate/2
  Product4/1 -> Sum4/1
  Product8/1 -> Sum7/1
  Product9/1 -> Sum9/1
  Selector4/1 -> Product3/1, Product2/1
  For Each Subsystem/1(Out1) -> i/1
  Signal Specification/1 -> For Each Subsystem/1(In1)
  Constant1/1 -> Matrix Concatenate/3
  Selector5/1 -> Product/2, Product1/1
  Selector8/1 -> Product6/2, Product7/1
  [omega_base] -> Selector8/1
  Gain5/1 -> Product6/1
  Gain6/1 -> Product7/2
  Product6/1 -> i_d/1
  Product7/1 -> i_q/1
  connected1/1 -> Selector6/1
  Selector/1 -> Product4/2
  Selector6/1 -> Product9/1, Product8/1, Product5/1, Product4/1
  Selector2/1 -> Product5/2
  Selector1/1 -> Product8/2
  Selector3/1 -> Product9/2

== system VFlexP/Grid/Grid/Dynamic/Lines/static ==
  v_in : Inport
  v_out_d : Inport  Port=2
  connected : Inport  Port=3
  Constant : Constant  Value=R_Lines(line_complexity == 2).^2  VectorParams1D=off
  Constant1 : Constant
  Constant2 : Constant  Value=zeros(1, sum(line_complexity == 2))  VectorParams1D=off
  Divide : Product  Inputs=*/
  For Each Subsystem : Subsystem  TreatAsAtomicUnit=on
  Gain : Gain  Gain=L_Lines(line_complexity == 2)
  Gain1 : Gain  Gain=R_Lines(line_complexity == 2)
  Gain2 : Gain  Gain=R_Lines(line_complexity == 2)
  Matrix Concatenate : Concatenate  NumInputs=3  Mode=Multidimensional array
  Product{,1..7} (8 alike) : Product
  Selector : Selector  NumberOfDimensions=2  InputPortWidth=3  IndexOptions=Index vector (dialog),Index vector (dialog)  Indices=1,find(line_complexity == 2)  OutputSizes=1,1
  Selector1 : Selector  NumberOfDimensions=2  InputPortWidth=3  IndexOptions=Index vector (dialog),Index vector (dialog)  Indices=1,find(line_complexity == 2)  OutputSizes=1,1
  Selector2 : Selector  NumberOfDimensions=2  InputPortWidth=3  IndexOptions=Index vector (dialog),Index vector (dialog)  Indices=2,find(line_complexity == 2)  OutputSizes=1,1
  Selector3 : Selector  NumberOfDimensions=2  InputPortWidth=3  IndexOptions=Index vector (dialog),Index vector (dialog)  Indices=2,find(line_complexity == 2)  OutputSizes=1,1
  Selector4 : Selector  InputPortWidth=length(From_buses)  IndexOptions=Index vector (dialog)  Indices=find(line_complexity == 2)  OutputSizes=1
  Selector5 : Selector  InputPortWidth=length(fref.ref_units)  IndexOptions=Index vector (dialog)  Indices=fref.lines(line_complexity == 2)  OutputSizes=1
  Sum : Sum  Inputs=|++
  Sum1 : Sum  Inputs=|+-
  Sum2 : Sum  Inputs=|+-
  Sum3 : Sum  Inputs=|++
  Sum4 : Sum  Inputs=|-+
  i : Outport
  wires:
  [omega_ref] -> Selector5/1  "omega"
  Sum4/1 -> Product7/2  "iq"
  Sum3/1 -> Product6/2  "id"
  Gain1/1 -> Product1/2
  Product2/1 -> Product4/2, Product3/1
  Product4/1 -> Sum4/1
  Divide/1 -> Gain2/1, Gain1/1, Product2/1
  Sum1/1 -> Product1/1, Product4/1  "vd"
  Product3/1 -> Sum3/2
  Constant1/1 -> Divide/1
  Gain/1 -> Product2/2, Product/2, Product/1
  Sum2/1 -> Product5/1, Product3/2  "vq"
  Constant/1 -> Sum/1
  Product5/1 -> Sum4/2
  Product1/1 -> Sum3/1
  Product/1 -> Sum/2
  Gain2/1 -> Product5/2
  Sum/1 -> Divide/2
  v_out_d/1 -> Selector3/1, Selector1/1  "v_out_d"
  v_in/1 -> Selector2/1, Selector/1
  connected/1 -> Selector4/1
  Selector1/1 -> Sum1/2
  Selector3/1 -> Sum2/2
  Selector2/1 -> Sum2/1
  Selector/1 -> Sum1/1
  Matrix Concatenate/1 -> For Each Subsystem/1(In1)
  Product6/1 -> Matrix Concatenate/1
  Product7/1 -> Matrix Concatenate/2
  Selector4/1 -> Product7/1, Product6/1
  For Each Subsystem/1(Out1) -> i/1
  Constant2/1 -> Matrix Concatenate/3
  Selector5/1 -> Gain/1

== system VFlexP/Grid/Grid/Dynamic/Lines/static omega ==
  v_in_d : Inport
  v_out : Inport  Port=2
  connected : Inport  Port=3
  Constant1 : Constant  Value=zeros(1, sum(line_complexity == 3))  VectorParams1D=off
  For Each Subsystem : Subsystem  TreatAsAtomicUnit=on
  Gain : Gain  Gain=1./(R_Lines(line_complexity == 3).^2+L_Lines(line_complexity == 3).^2)
  Gain1 : Gain  Gain=1./(R_Lines(line_complexity == 3).^2+L_Lines(line_complexity == 3).^2)
  Gain3 : Gain  Gain=R_Lines(line_complexity == 3)
  Gain4 : Gain  Gain=L_Lines(line_complexity == 3)
  Gain5 : Gain  Gain=L_Lines(line_complexity == 3)
  Gain6 : Gain  Gain=R_Lines(line_complexity == 3)
  Matrix Concatenate : Concatenate  NumInputs=3  Mode=Multidimensional array
  Product2 : Product
  Product3 : Product
  Selector : Selector  NumberOfDimensions=2  InputPortWidth=3  IndexOptions=Index vector (dialog),Index vector (dialog)  Indices=1,find(line_complexity == 3)  OutputSizes=1,1
  Selector1 : Selector  NumberOfDimensions=2  InputPortWidth=3  IndexOptions=Index vector (dialog),Index vector (dialog)  Indices=1,find(line_complexity == 3)  OutputSizes=1,1
  Selector2 : Selector  NumberOfDimensions=2  InputPortWidth=3  IndexOptions=Index vector (dialog),Index vector (dialog)  Indices=2,find(line_complexity == 3)  OutputSizes=1,1
  Selector3 : Selector  NumberOfDimensions=2  InputPortWidth=3  IndexOptions=Index vector (dialog),Index vector (dialog)  Indices=2,find(line_complexity == 3)  OutputSizes=1,1
  Selector4 : Selector  InputPortWidth=length(From_buses)  IndexOptions=Index vector (dialog)  Indices=find(line_complexity == 3)  OutputSizes=1
  Sum : Sum  Inputs=|++
  Sum1 : Sum  Inputs=|+-
  Sum2 : Sum  Inputs=|+-
  Sum3 : Sum  Inputs=|-+
  i : Outport
  wires:
  Selector3/1 -> Sum2/2  "v_out_q"
  Sum1/1 -> Gain/1  "vd"
  Sum2/1 -> Gain1/1  "vq"
  Gain/1 -> Gain3/1, Gain5/1
  Gain3/1 -> Sum/1
  Gain4/1 -> Sum/2
  Gain1/1 -> Gain4/1, Gain6/1
  Sum/1 -> Product2/2
  Gain5/1 -> Sum3/1
  Sum3/1 -> Product3/2
  Gain6/1 -> Sum3/2
  connected/1 -> Selector4/1
  Matrix Concatenate/1 -> For Each Subsystem/1(In1)
  Product2/1 -> Matrix Concatenate/1
  Product3/1 -> Matrix Concatenate/2
  v_in_d/1 -> Selector2/1, Selector/1  "v_in"
  Selector/1 -> Sum1/1
  Selector2/1 -> Sum2/1
  v_out/1 -> Selector3/1, Selector1/1
  Selector1/1 -> Sum1/2
  Selector4/1 -> Product3/1, Product2/1
  For Each Subsystem/1(Out1) -> i/1
  Constant1/1 -> Matrix Concatenate/3

== system VFlexP/Grid/Grid/Dynamic/Lines/tap transformer ==
  in_d : Inport
  in_q : Inport  Port=2
  Complex to Real-Imag : ComplexToRealImag
  Gain : Gain  Gain=1./tap_lines.*(cos(shift_lines)-1i*sin(shift_lines))
  Real-Imag to Complex : RealImagToComplex
  out_d : Outport
  out_q : Outport  Port=2
  wires:
  Complex to Real-Imag/2 -> out_q/1
  Real-Imag to Complex/1 -> Gain/1
  Gain/1 -> Complex to Real-Imag/1
  Complex to Real-Imag/1 -> out_d/1
  in_q/1 -> Real-Imag to Complex/2
  in_d/1 -> Real-Imag to Complex/1

== system VFlexP/Grid/Grid/Dynamic/Lines to buses/Lines_toM ==
  i_to : Inport  Partition=on  PartitionDimension=1  PartitionWidth=1  PartitionOffset=0
  i_from : Inport  Port=2  Partition=on  PartitionDimension=1  PartitionWidth=1  PartitionOffset=0
  For Each : ForEach  DisableCoverage=on
  State-Space : StateSpace  A=[]  B=[]  C=[]  D=Lines_toM  InitialCondition=0  ParameterTunability=Optimized
  State-Space1 : StateSpace  A=[]  B=[]  C=[]  D=Lines_fromM  InitialCondition=0  ParameterTunability=Optimized
  Transpose{,1..3} (4 alike) : Math  Operator=transpose
  i_from_lines : Outport  ConcatenationDimension=1
  i_to_lines : Outport  Port=2  ConcatenationDimension=1
  wires:
  Transpose1/1 -> i_from_lines/1
  i_to/1 -> Transpose/1
  State-Space/1 -> Transpose1/1
  Transpose/1 -> State-Space/1
  Transpose2/1 -> State-Space1/1
  State-Space1/1 -> Transpose3/1
  i_from/1 -> Transpose2/1
  Transpose3/1 -> i_to_lines/1

== system VFlexP/Grid/Grid/Dynamic/Loads/PQ ==
  v_in : Inport
  connected : Inport  Port=2
  iP : Inport  Port=3
  Constant : Constant  Value=Ploads(load_complexity == 4)/Sb  VectorParams1D=off
  Constant1 : Constant  Value=Qloads(load_complexity == 4)/Sb  VectorParams1D=off
  Constant2 : Constant  Value=Inf
  Constant3 : Constant  Value=zeros(1, sum(load_complexity == 4))  VectorParams1D=off
  Divide : Product  Inputs=*/
  Divide1 : Product  Inputs=*/
  For Each Subsystem : Subsystem  TreatAsAtomicUnit=on
  Gain : Gain  Gain=Ploads(load_complexity == 4)/Sb
  Matrix Concatenate : Concatenate  NumInputs=3  Mode=Multidimensional array
  Product{,1..7} (8 alike) : Product
  Selector : Selector  NumberOfDimensions=2  InputPortWidth=3  IndexOptions=Index vector (dialog),Index vector (dialog)  Indices=1,find(load_complexity == 4)  OutputSizes=1,1
  Selector1 : Selector  NumberOfDimensions=2  InputPortWidth=3  IndexOptions=Index vector (dialog),Index vector (dialog)  Indices=2,find(load_complexity == 4)  OutputSizes=1,1
  Selector2 : Selector  InputPortWidth=length(R_Loads)  IndexOptions=Index vector (dialog)  Indices=find(load_complexity == 4)  OutputSizes=1
  Selector3 : Selector  InputPortWidth=length(R_Loads)  IndexOptions=Index vector (dialog)  Indices=find(load_complexity == 4)  OutputSizes=1
  Sum : Sum  Inputs=|++
  Sum1 : Sum  Inputs=|+-
  Sum2 : Sum  Inputs=|++
  Sum4 : Sum  Inputs=|++
  Switch : Switch  Criteria=u2 > Threshold  Threshold=1e-5  ZeroCross=off  SaturateOnIntegerOverflow=off  InputSameDT=off
  i : Outport
  wires:
  Product1/1 -> Sum/2
  Product/1 -> Sum/1
  Sum2/1 -> Product/1, Product2/1  "Prefnew"
  Product2/1 -> Sum1/1
  v_in/1 -> Selector1/1, Selector/1
  Product3/1 -> Sum1/2
  Product5/1 -> Sum4/2
  Constant1/1 -> Product3/1, Product1/2  "Qrefnew"
  Product4/1 -> Sum4/1
  Sum/1 -> Divide/1
  Switch/1 -> Divide1/2, Divide/2
  Sum4/1 -> Switch/1, Switch/2
  Constant2/1 -> Switch/3
  Sum1/1 -> Divide1/1
  connected/1 -> Selector2/1
  Divide/1 -> Product6/2  "id"
  Divide1/1 -> Product7/2  "iqref"
  Selector/1 -> Product4/1, Product4/2, Product/2, Product3/2  "id1"
  Selector1/1 -> Product5/1, Product5/2, Product2/2, Product1/1  "iq1"
  Matrix Concatenate/1 -> For Each Subsystem/1(In1)
  Product6/1 -> Matrix Concatenate/1
  Product7/1 -> Matrix Concatenate/2
  Selector2/1 -> Product6/1, Product7/1
  For Each Subsystem/1(Out1) -> i/1
  Constant3/1 -> Matrix Concatenate/3
  Selector3/1 -> Gain/1
  Gain/1 -> Sum2/1
  iP/1 -> Selector3/1
  Constant/1 -> Sum2/2  "Prefnew"
